simulink model "ModelareMasina"  (R2018a)
settings: Solver=VariableStepAuto  StartTime=0.0  StopTime=10.0  RelTol=1e-3  EnableMultiTasking=on
values from neighbouring files (symbols this model uses):
  brk = 0.65    [BuggatiVeyron.mat]    (also in Duster.mat)
  frCfn = 0.97    [BuggatiVeyron.mat]    (also in Duster.mat = 0.2)
  grAcc = 9.81    [BuggatiVeyron.mat]    (also in Duster.mat)
  mass = 1950.447191    [BuggatiVeyron.mat]    (also in Duster.mat = 1395)
  pow = 1118549.808    [BuggatiVeyron.mat]    (also in Duster.mat = 62489.649274)
  rTime = 1.35    [BuggatiVeyron.mat]    (also in Duster.mat)
settings Model: Creator=novac  LastModifiedBy=Paul
settings OptimizationCC: LifeSpan=inf
settings DebuggingCC: SFUnexpectedBacktrackingDiag=warning  SFNoUnconditionalDefaultTransitionDiag=warning  SFExecutionAtInitializationDiag=none
settings CodeAppCC: StateflowObjectComments=on
settings GRTTargetCC: TargetLangStandard=C89/C90 (ANSI)  GeneratePreprocessorConditionals=Disable all
settings ConfigComp: CovMetricSettings=dw  CovHtmlReporting=on  CovSaveCumulativeToWorkspaceVar=on  CovSaveSingleToWorkspaceVar=on  CovExternalEMLEnable=off

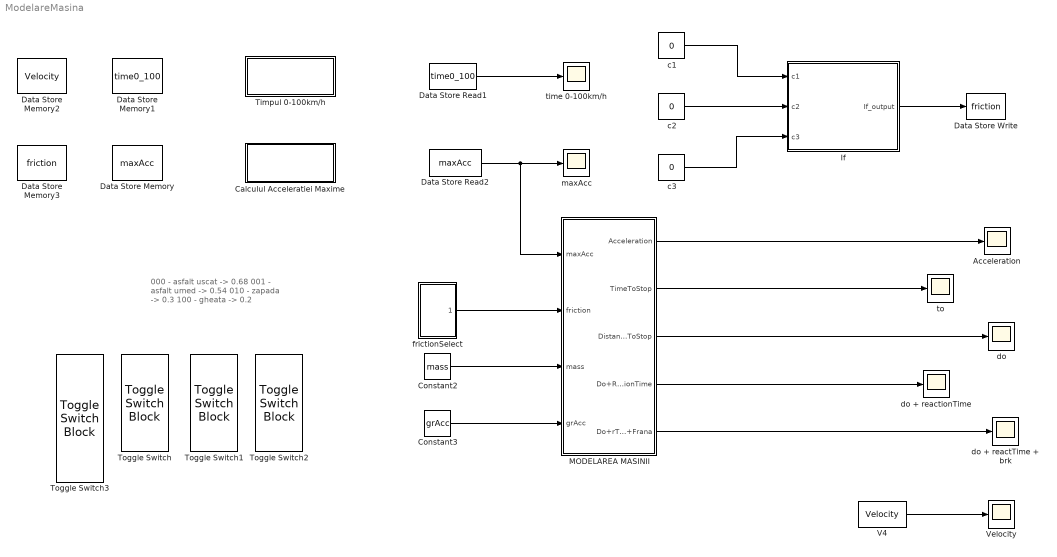
== system ModelareMasina ==
  note: 000 - asfalt uscat -> 0.68
      | 001 - asfalt umed -> 0.54
      | 010 - zapada -> 0.3
      | 100 - gheata -> 0.2
  Acceleration : Scope
  Calculul Acceleratiei Maxime : Subsystem  TreatAsAtomicUnit=on
  Constant2 : Constant  Value=mass
  Constant3 : Constant  Value=grAcc
  Data Store Memory : DataStoreMemory  DataStoreName=maxAcc  ReadBeforeWriteMsg=warning  WriteAfterWriteMsg=warning  WriteAfterReadMsg=warning  ShowAdditionalParam=off
  Data Store Memory1 : DataStoreMemory  DataStoreName=time0_100  ReadBeforeWriteMsg=warning  WriteAfterWriteMsg=warning  WriteAfterReadMsg=warning  ShowAdditionalParam=off
  Data Store Memory2 : DataStoreMemory  DataStoreName=Velocity  ReadBeforeWriteMsg=warning  WriteAfterWriteMsg=warning  WriteAfterReadMsg=warning  ShowAdditionalParam=off
  Data Store Memory3 : DataStoreMemory  DataStoreName=friction  ReadBeforeWriteMsg=warning  WriteAfterWriteMsg=warning  WriteAfterReadMsg=warning  ShowAdditionalParam=off
  Data Store Read1 : DataStoreRead  DataStoreName=time0_100
  Data Store Read2 : DataStoreRead  DataStoreName=maxAcc
  Data Store Write : DataStoreWrite  DataStoreName=friction
  If : Stateflow chart  TreatAsAtomicUnit=on
  MODELAREA MASINII : Subsystem
  Timpul 0-100km/h : Subsystem  TreatAsAtomicUnit=on
  Toggle Switch : ToggleSwitchBlock  WebBlockId=186  LabelPosition=Hide
      settings: Values={{'Off', 'On'}, [0 1]}
  Toggle Switch1 : ToggleSwitchBlock  WebBlockId=184  LabelPosition=Hide
      settings: Values={{'Off', 'On'}, [0 1]}
  Toggle Switch2 : ToggleSwitchBlock  WebBlockId=183  LabelPosition=Hide
      settings: Values={{'Off', 'On'}, [0 1]}
  Toggle Switch3 : ToggleSwitchBlock  WebBlockId=185  LabelPosition=Bottom
      settings: Values={{'Off', 'On'}, [0 1]}
  V4 : DataStoreRead  DataStoreName=Velocity
  Velocity : Scope
  c1 : Constant  Value=0
  c2 : Constant  Value=0
  c3 : Constant  Value=0
  do : Scope
  do + reactTime + brk : Scope
  do + reactionTime : Scope
  frictionSelect : Subsystem
  maxAcc : Scope
  time 0-100km/h : Scope
  to : Scope
  wires:
  Data Store Read1/1 -> time 0-100km/h/1
  Data Store Read2/1 -> MODELAREA MASINII/1(maxAcc), maxAcc/1
  If/1(If_output) -> Data Store Write/1
  c1/1 -> If/1(c1)
  c2/1 -> If/2(c2)
  c3/1 -> If/3(c3)
  V4/1 -> Velocity/1
  frictionSelect/1(friction) -> MODELAREA MASINII/2(friction)
  Constant2/1 -> MODELAREA MASINII/3(mass)
  Constant3/1 -> MODELAREA MASINII/4(grAcc)
  MODELAREA MASINII/1(Acceleration) -> Acceleration/1
  MODELAREA MASINII/2(TimeToStop) -> to/1
  MODELAREA MASINII/3(DistanceToStop) -> do/1
  MODELAREA MASINII/4(Do+ReactionTime) -> do + reactionTime/1
  MODELAREA MASINII/5(Do+rTime+Frana) -> do + reactTime + brk/1

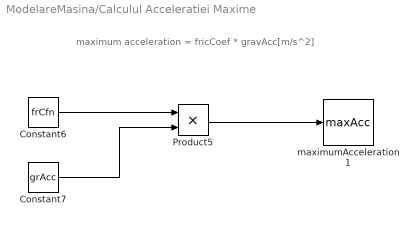
== system ModelareMasina/Calculul Acceleratiei Maxime ==
  note: maximum acceleration = fricCoef * gravAcc[m/s^2]
  Constant6 : Constant  Value=frCfn
  Constant7 : Constant  Value=grAcc
  Product5 : Product
  maximumAcceleration1 : DataStoreWrite  DataStoreName=maxAcc
  wires:
  Constant6/1 -> Product5/1
  Constant7/1 -> Product5/2
  Product5/1 -> maximumAcceleration1/1

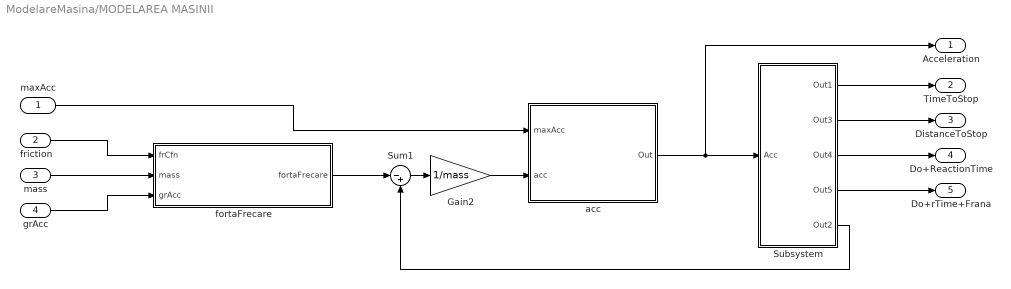
== system ModelareMasina/MODELAREA MASINII ==
  maxAcc : Inport
  friction : Inport  Port=2
  mass : Inport  Port=3
  grAcc : Inport  Port=4
  Gain2 : Gain  Gain=1/mass
  Subsystem : Subsystem
  Sum1 : Sum  Inputs=|-+
  acc : Stateflow chart  TreatAsAtomicUnit=on
  fortaFrecare : Subsystem
  Acceleration : Outport
  TimeToStop : Outport  Port=2
  DistanceToStop : Outport  Port=3
  Do+ReactionTime : Outport  Port=4
  Do+rTime+Frana : Outport  Port=5
  wires:
  acc/1(Out) -> Acceleration/1, Subsystem/1(Acc)
  Gain2/1 -> acc/2(acc)
  Sum1/1 -> Gain2/1
  grAcc/1 -> fortaFrecare/3(" grAcc")
  mass/1 -> fortaFrecare/2(mass)
  friction/1 -> fortaFrecare/1(frCfn)
  fortaFrecare/1(fortaFrecare) -> Sum1/1
  maxAcc/1 -> acc/1(maxAcc)
  Subsystem/4(Out5) -> Do+rTime+Frana/1
  Subsystem/2(Out3) -> DistanceToStop/1
  Subsystem/1(Out1) -> TimeToStop/1
  Subsystem/5(Out2) -> Sum1/2
  Subsystem/3(Out4) -> Do+ReactionTime/1

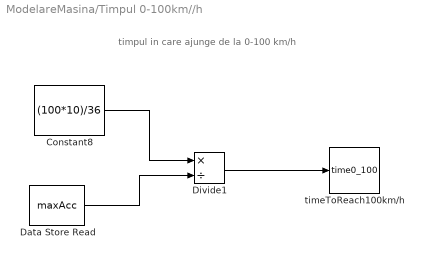
== system ModelareMasina/Timpul 0-100km//h ==
  note: timpul in care ajunge de la 0-100 km/h
  Constant8 : Constant  Value=(100*10)/36
  Data Store Read : DataStoreRead  DataStoreName=maxAcc
  Divide1 : Product  Inputs=*/
  timeToReach100km/h : DataStoreWrite  DataStoreName=time0_100
  wires:
  Constant8/1 -> Divide1/1
  Data Store Read/1 -> Divide1/2
  Divide1/1 -> timeToReach100km/h/1

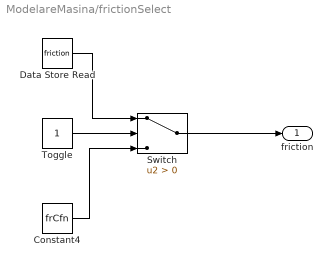
== system ModelareMasina/frictionSelect ==
  Constant4 : Constant  Value=frCfn
  Data Store Read : DataStoreRead  DataStoreName=friction
  Switch : Switch  Criteria=u2 > Threshold
  "Toggle " : Constant
  friction : Outport
  wires:
  "Toggle "/1 -> Switch/2
  Constant4/1 -> Switch/3
  Switch/1 -> friction/1
  Data Store Read/1 -> Switch/1

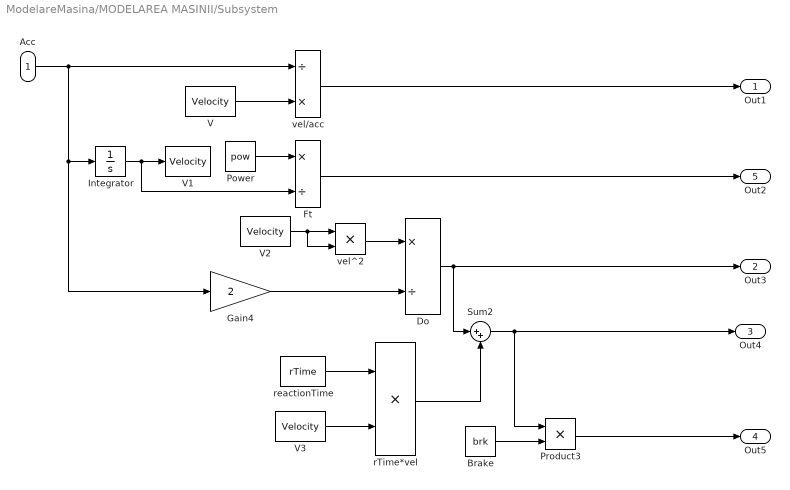
== system ModelareMasina/MODELAREA MASINII/Subsystem ==
  Acc : Inport
  Brake : Constant  Value=brk
  Do : Product  Inputs=*/
  Ft : Product  Inputs=*/
  Gain4 : Gain  Gain=2
  Integrator : Integrator  InitialCondition=10
  Power : Constant  Value=pow
  Product3 : Product
  Sum2 : Sum  Inputs=|++
  V : DataStoreRead  DataStoreName=Velocity
  V1 : DataStoreWrite  DataStoreName=Velocity
  V2 : DataStoreRead  DataStoreName=Velocity
  V3 : DataStoreRead  DataStoreName=Velocity
  rTime*vel : Product
  reactionTime : Constant  Value=rTime
  vel/acc : Product  Inputs=/*
  vel^2 : Product
  Out1 : Outport
  Out3 : Outport  Port=2
  Out4 : Outport  Port=3
  Out5 : Outport  Port=4
  Out2 : Outport  Port=5
  wires:
  Ft/1 -> Out2/1
  Power/1 -> Ft/1
  vel^2/1 -> Do/1
  vel/acc/1 -> Out1/1
  Integrator/1 -> V1/1, Ft/2
  Sum2/1 -> Out4/1, Product3/1
  Gain4/1 -> Do/2
  reactionTime/1 -> rTime*vel/1
  Product3/1 -> Out5/1
  Do/1 -> Sum2/1, Out3/1
  rTime*vel/1 -> Sum2/2
  Brake/1 -> Product3/2
  V3/1 -> rTime*vel/2
  V/1 -> vel/acc/2
  Acc/1 -> Integrator/1, Gain4/1, vel/acc/1
  V2/1 -> vel^2/2, vel^2/1

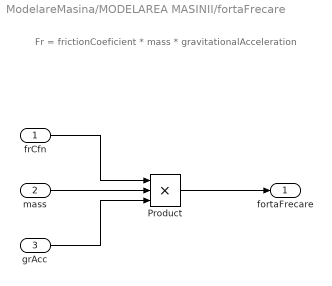
== system ModelareMasina/MODELAREA MASINII/fortaFrecare ==
  note: Fr = frictionCoeficient * mass * gravitationalAcceleration
  frCfn : Inport
  mass : Inport  Port=2
  " grAcc" : Inport  Port=3
  Product : Product  Inputs=3
  fortaFrecare : Outport
  wires:
  frCfn/1 -> Product/1
  mass/1 -> Product/2
  " grAcc"/1 -> Product/3
  Product/1 -> fortaFrecare/1

== stateflow chart ModelareMasina/MODELAREA MASINII/acc ==
  note: Equivalent M-Code:
      |
      | if maxAcc >= acc
      |     Out = acc;
      | else
      |    Out = maxAcc;
      | end
  (default) -> (junction 12)
  (junction 12) -> (junction 15) [order 1] : [maxAcc>=acc]
  (junction 12) -> (junction 13) [order 2] : {Out=maxAcc;}
  (junction 15) -> (junction 13) : {Out=acc;}
  data: maxAcc input double; Out output double; acc input

== stateflow chart ModelareMasina/If ==
  (default) -> (junction 12)
  (junction 12) -> (junction 15) [order 1] : [c1 == 0 & c2 == 0 & c3 == 0]
  (junction 15) -> (junction 38) : {If_output=0.68;}
  (junction 12) -> (junction 14) [order 2]
  (junction 14) -> (junction 17) [order 1] : [c1 == 0 & c2 == 0 & c3 == 1]
  (junction 17) -> (junction 37) : {If_output=0.54}
  (junction 14) -> (junction 19) [order 2]
  (junction 19) -> (junction 32) [order 1] : [c1 == 0 & c2 == 1 & c3 == 0]
  (junction 32) -> (junction 34) : {If_output=0.3;}
  (junction 19) -> (junction 43) [order 2] : {If_output=0.2;}
  (junction 34) -> (junction 43)
  (junction 37) -> (junction 34)
  (junction 38) -> (junction 37)
  (junction 43) -> (junction 46)
  data: If_output output double; c1 input; c2 input; c3 input
